simulink model "H2"  (Simulink 7.3)
settings: Solver=ode23  StartTime=0.0  StopTime=2  RelTol=1e-4
settings Model: Creator=Admin  LastModifiedBy=Sainquake Notebook
settings DebuggingCC: StrictBusMsg=ErrorLevel1

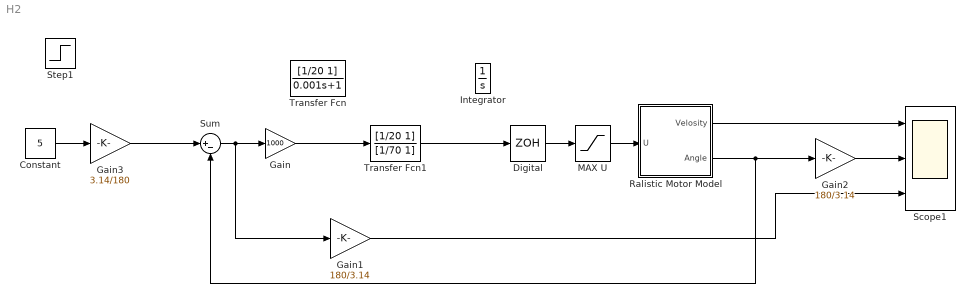
== system H2 ==
  Constant : Constant  Value=5  OutDataType=fixdt(1, 16)  OutScaling=2^0
  Digital : ZeroOrderHold  SampleTime=1/19531.25
  Gain : Gain  Gain=1000  ParameterDataType=fixdt(1, 16)  ParameterScaling=2^0  OutDataType=fixdt(1, 16)  OutScaling=2^0
  Gain1 : Gain  Gain=180/3.14  ParameterDataType=fixdt(1, 16)  ParameterScaling=2^0  OutDataType=fixdt(1, 16)  OutScaling=2^0
  Gain2 : Gain  Gain=180/3.14  ParameterDataType=fixdt(1, 16)  ParameterScaling=2^0  OutDataType=fixdt(1, 16)  OutScaling=2^0
  Gain3 : Gain  Gain=3.14/180  ParameterDataType=fixdt(1, 16)  ParameterScaling=2^0  OutDataType=fixdt(1, 16)  OutScaling=2^0
  Integrator : Integrator
  MAX U : Saturate  UpperLimit=27  LowerLimit=-27
  Ralistic Motor Model : Subsystem  TreatAsAtomicUnit=on
  Scope1 : Scope  NumInputPorts=3
      settings: YMin=5e-005~5.0205~-0.02425  YMax=0.0003~5.02425~-0.0205  MaxDataPoints=500000
  Step1 : Step  Time=5  After=-20  SampleTime=0
  Sum : Sum  Inputs=|+-  OutDataType=fixdt(1, 16)  OutScaling=2^0
  Transfer Fcn : TransferFcn  Numerator=[1/20 1]  Denominator=[0.001 1]
  Transfer Fcn1 : TransferFcn  Numerator=[1/20 1]  Denominator=[1/70 1]
  wires:
  MAX U/1 -> Ralistic Motor Model/1(U)
  Digital/1 -> MAX U/1
  Ralistic Motor Model/1(Velosity) -> Scope1/1
  Ralistic Motor Model/2(Angle) -> Sum/2, Gain2/1
  Sum/1 -> Gain/1, Gain1/1
  Constant/1 -> Gain3/1
  Gain/1 -> Transfer Fcn1/1
  Transfer Fcn1/1 -> Digital/1
  Gain1/1 -> Scope1/3
  Gain2/1 -> Scope1/2
  Gain3/1 -> Sum/1

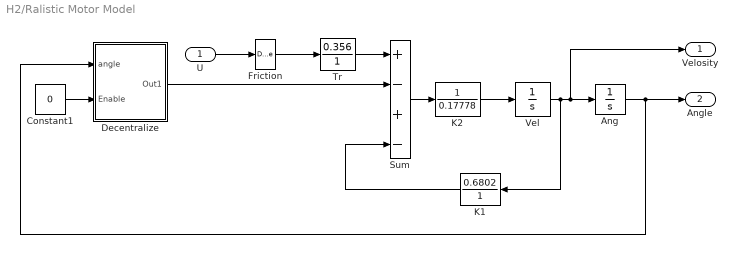
== system H2/Ralistic Motor Model ==
  U : Inport  OutDataType=fixdt(1, 16)  OutScaling=2^0
  Ang : Integrator
  Constant1 : Constant  Value=0  OutDataType=fixdt(1, 16)  OutScaling=2^0
  Decentralize : Subsystem  TreatAsAtomicUnit=on
  Friction : DeadZone  LowerValue=-1.4  UpperValue=1.4  SaturateOnIntegerOverflow=on
  K1 : TransferFcn  Numerator=[0.6802]  Denominator=[ 1]
  K2 : TransferFcn  Denominator=0.17778
  Sum : Sum  Inputs=+-+-
  Tr : TransferFcn  Numerator=[0.356]  Denominator=[ 1 ]
  Vel : Integrator
  Velosity : Outport  OutDataType=fixdt(1, 16)  OutScaling=2^0
  Angle : Outport  Port=2  OutDataType=fixdt(1, 16)  OutScaling=2^0
  wires:
  Sum/1 -> K2/1
  K2/1 -> Vel/1
  Ang/1 -> Decentralize/1(angle), Angle/1
  K1/1 -> Sum/4
  Tr/1 -> Sum/1
  Decentralize/1(Out1) -> Sum/2
  Friction/1 -> Tr/1
  U/1 -> Friction/1
  Constant1/1 -> Decentralize/2(Enable)
  Vel/1 -> K1/1, Ang/1, Velosity/1

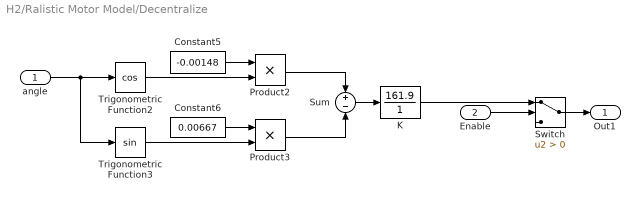
== system H2/Ralistic Motor Model/Decentralize ==
  angle : Inport  OutDataType=fixdt(1, 16)  OutScaling=2^0
  Enable : Inport  Port=2  OutDataType=fixdt(1, 16)  OutScaling=2^0
  Constant5 : Constant  Value=-0.00148
  Constant6 : Constant  Value=0.00667
  K : TransferFcn  Numerator=[161.9]  Denominator=[ 1 ]
  Product2 : Product  RndMeth=Zero
  Product3 : Product  RndMeth=Zero
  Sum : Sum  Inputs=+|-  OutDataType=fixdt(1, 16)  OutScaling=2^0
  Switch : Switch  Criteria=u2 > Threshold  OutDataType=fixdt(1, 16)  OutScaling=2^0
  Trigonometric Function2 : Trigonometry  Operator=cos
  Trigonometric Function3 : Trigonometry
  Out1 : Outport  OutDataType=fixdt(1, 16)  OutScaling=2^0
  wires:
  Constant5/1 -> Product2/1
  Trigonometric Function2/1 -> Product2/2
  Constant6/1 -> Product3/1
  Trigonometric Function3/1 -> Product3/2
  Product3/1 -> Sum/2
  Product2/1 -> Sum/1
  Sum/1 -> K/1
  K/1 -> Switch/1
  angle/1 -> Trigonometric Function2/1, Trigonometric Function3/1
  Enable/1 -> Switch/2
  Switch/1 -> Out1/1
